simulink model "digrama_bloques"  (R2021a)
settings: Solver=VariableStepAuto  StartTime=0.0  StopTime=20.0  RelTol=1e-3
values from neighbouring files (symbols this model uses):
  G = tf([0.4 2],conv([3 1],[1 1]))    [preg2.m]    (also in preg4.m = 1/(s*(s+1)*(s+2)); test.m = 2/(3*s+1)/(s+1))
settings Model: Creator=pierr  LastModifiedBy=pierr

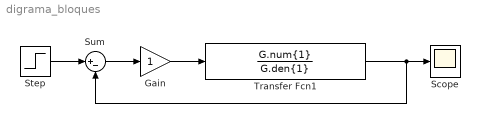
== system digrama_bloques ==
  Gain : Gain
  Scope : Scope
  Step : Step  SampleTime=0
  Sum : Sum  Inputs=|+-
  Transfer Fcn1 : TransferFcn  Numerator=G.num{1}  Denominator=G.den{1}
  wires:
  Transfer Fcn1/1 -> Sum/2, Scope/1
  Step/1 -> Sum/1
  Sum/1 -> Gain/1
  Gain/1 -> Transfer Fcn1/1
